simulink model "simple_circuits"  (R2024b)
settings: Solver=VariableStepAuto  StartTime=0.0  StopTime=10.0  RelTol=1e-3
libraries: spsRMSLib x4, spsSeriesRLCBranchLib x4, spsVoltageMeasurementLib x4, spsCurrentMeasurementLib x2, spsMultimeterLib x2, spsACVoltageSourceLib x1, spsDCVoltageSourceLib x1, sps_lib x1
settings Model: Creator=sanja  LastModifiedBy=sanja

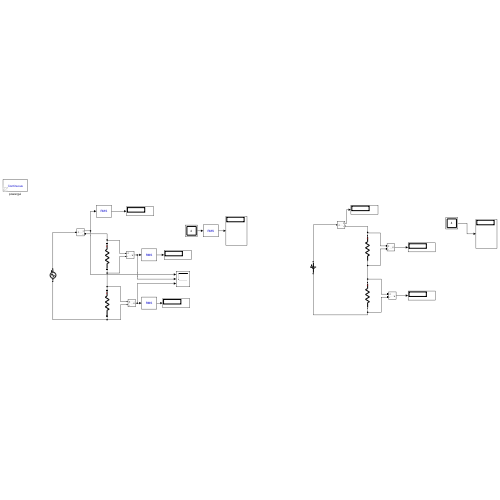
[thumbnail: Simulink's stored preview of the top-level diagram]
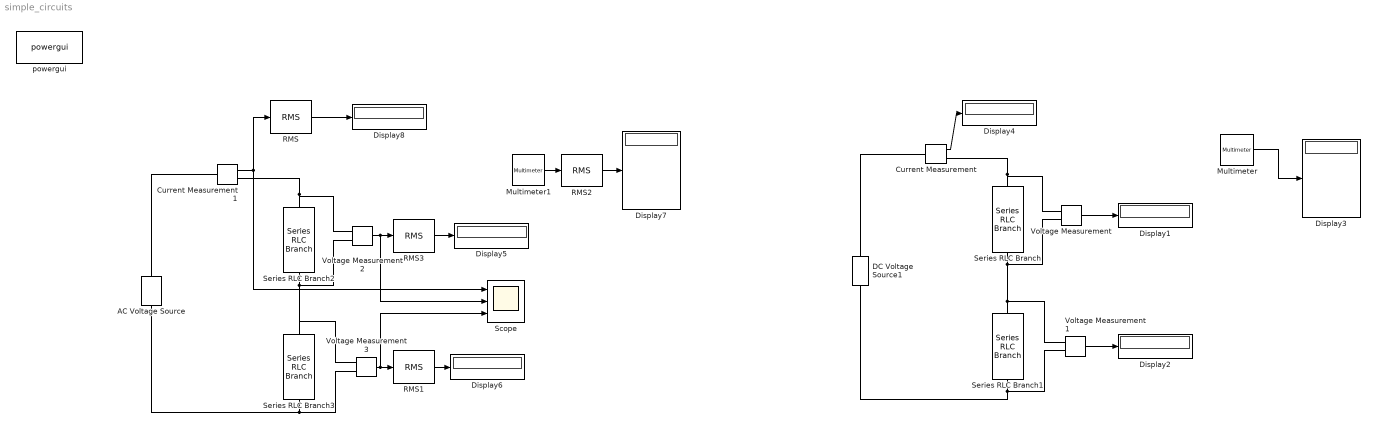
== system simple_circuits ==
  AC Voltage Source : spsACVoltageSourceLib/AC Voltage Source  Amplitude=220  Phase=0  Frequency=50  SampleTime=0  Measurements=None  BusType=swing  Pref=10e3  Qref=0  Qmin=-inf  Qmax=+inf
  Current Measurement : spsCurrentMeasurementLib/Current Measurement  PhasorSimulation=off  OutputType=Complex  PSBequivalent=0
  Current Measurement1 : spsCurrentMeasurementLib/Current Measurement  PhasorSimulation=off  OutputType=Complex  PSBequivalent=0
  DC Voltage Source1 : spsDCVoltageSourceLib/DC Voltage Source  Amplitude=50  Measurements=None
  Display{1..8} (8 alike) : Display
  Multimeter : spsMultimeterLib/Multimeter  L=8  sel=[1 2 5 6]  yselected={}  Gain=[1 1 1 1]  OutputType=Complex  PlotAtSimulationStop=off  PhasorSimulation=off
  Multimeter1 : spsMultimeterLib/Multimeter  L=8  sel=[3 4 7 8]  yselected={}  Gain=[1 1 1 1]  OutputType=Complex  PlotAtSimulationStop=on  PhasorSimulation=off
  RMS{,1..3} (4 alike) : spsRMSLib/RMS  TrueRMS=on  Freq=60  RMSInit=120  Ts=0
  Scope : Scope  NumInputPorts=3
  Series RLC Branch : spsSeriesRLCBranchLib/Series RLC Branch  LConnTagsString=__new0  RConnTagsString=__new0  BranchType=R  Resistance=10  Inductance=1e-3  SetiL0=off  InitialCurrent=0  Capacitance=1e-6  Setx0=off  InitialVoltage=0  Measurements=Branch voltage and current
  Series RLC Branch1 : spsSeriesRLCBranchLib/Series RLC Branch  LConnTagsString=__new0  RConnTagsString=__new0  BranchType=R  Resistance=5  Inductance=1e-3  SetiL0=off  InitialCurrent=0  Capacitance=1e-6  Setx0=off  InitialVoltage=0  Measurements=Branch voltage and current
  Series RLC Branch2 : spsSeriesRLCBranchLib/Series RLC Branch  LConnTagsString=__new0  RConnTagsString=__new0  BranchType=R  Resistance=10  Inductance=1e-3  SetiL0=off  InitialCurrent=0  Capacitance=1e-6  Setx0=off  InitialVoltage=0  Measurements=Branch voltage and current
  Series RLC Branch3 : spsSeriesRLCBranchLib/Series RLC Branch  LConnTagsString=__new0  RConnTagsString=__new0  BranchType=R  Resistance=5  Inductance=1e-3  SetiL0=off  InitialCurrent=0  Capacitance=1e-6  Setx0=off  InitialVoltage=0  Measurements=Branch voltage and current
  Voltage Measurement{,1..3} (4 alike) : spsVoltageMeasurementLib/Voltage Measurement  PhasorSimulation=off  OutputType=Complex  PSBequivalent=0
  powergui : sps_lib/powergui  Priority=1  SimulationMode=Continuous  SampleTime=50e-6  frequency=60  Iterations=50  frequencyindice=0  Pbase=100e6  ErrMax=1e-4  UnitsV=kV  UnitsW=MW  buscounter=0  FunctionMessages=off  echomessages=off  EnableUseOfTLC=off  CurrentSourceSwitches=off  DisableSnubberDevices=off  DisableRonSwitches=off  DisableVfSwitches=off  DisplayEquations=off  AutomaticDiscreteSolvers=off  SolverType=Tustin/Backward Euler (TBE)  Interpol=off  ExternalGateDelay=off  methode=off  Ts=100  x0status=blocks  SPID=on  SwTol=0  HookPort=off  NonlinearTolerance=1e-4  nMaxIteration=100  ContinueOnMaxIteration=off  RestoreLinks=warning  ResistiveCurrentMeasurement=off  Frange=[0:2:500]  Ylog=off  Xlog=on  ShowGrid=off  save=off  variable=ZData  structure=0  ZoomFFT=off  StartTime=0.0  cycles=1  DisplayStyle=1  fundamental=60  FreqAxis=off  MaxFrequency=1000  frequencyindicesteady=1  RmsSteady=1  display=off
  wires:
  Current Measurement/1 -> Display4/1
  Voltage Measurement/1 -> Display1/1
  Voltage Measurement1/1 -> Display2/1
  Multimeter/1 -> Display3/1
  Voltage Measurement2/1 -> Scope/2, RMS3/1
  Voltage Measurement3/1 -> Scope/3, RMS1/1
  Multimeter1/1 -> RMS2/1
  Current Measurement1/1 -> Scope/1, RMS/1
  RMS/1 -> Display8/1
  RMS3/1 -> Display5/1
  RMS1/1 -> Display6/1
  RMS2/1 -> Display7/1
  connections:
  Series RLC Branch1/LConn1 -- Voltage Measurement1/LConn1 -- Voltage Measurement/LConn2 -- Series RLC Branch/RConn1
  DC Voltage Source1/RConn1 -- Current Measurement/LConn1
  Series RLC Branch1/RConn1 -- Voltage Measurement1/LConn2 -- DC Voltage Source1/LConn1
  Current Measurement/RConn1 -- Voltage Measurement/LConn1 -- Series RLC Branch/LConn1
  Series RLC Branch2/LConn1 -- Current Measurement1/RConn1 -- Voltage Measurement2/LConn1
  Series RLC Branch2/RConn1 -- Voltage Measurement3/LConn1 -- Series RLC Branch3/LConn1 -- Voltage Measurement2/LConn2
  Series RLC Branch3/RConn1 -- AC Voltage Source/LConn1 -- Voltage Measurement3/LConn2
  AC Voltage Source/RConn1 -- Current Measurement1/LConn1
